simulink model "aIEEE13bus_with_solar_13bus_pl_1day"  (R2025a)
settings: Solver=ode4  StartTime=0.0  StopTime=168  FixedStep=5e-6  MaxStep=1e-4  RelTol=1e-4
InitFcn:
  | a=1; % Loading Factor
  | Ts=50e-6;
  | % phase to sequence conversion of RXB matrices
  | c=1*exp(sqrt(-1)*(120*pi/180));
  | T=[1 1 1;1 c*c c;1 c c*c];
  | Tinv=1/3*[1 1 1;1 c c*c;1 c*c c];
  | 
  | % Simulation data for the IEEE 13 Node Test Feeder model
  | mi2km = 1.60934;%  miles to km conversion
  | ft2km = 0.0003048; % feet to km conversion
  | ms2F = 1*1e-6/(2*pi*60);% microsiemens to Farads conversion
  | 
  | 
  | %% Configuration 601
  | % Series Resitance and Reactance - ohm/mile
  | R_601 = [0.3465 0.1560 0.1580;0.1560 0.3375 0.1535;0.1580 0.1535 0.3414];
  | X_601 = [1.1079 0.5017 0.4236;0.5017 1.0478 0.3849;0.4236 0.3849 1.0348];
  | % charging susceptance - microsiemens/mile
  | B_601 = [6.2998 -1.9958 -1.2595;-1.9958 5.9597 -0.7417;-1.2595 -0.7417 5.6386];
  | 
  | R_601 = R_601/mi2km;
  | Rseq=Tinv*R_601*T;
  | R1_601=Rseq(2,2);R0_601=Rseq(1,1);
  | 
  | L_601 = (X_601/(2*pi*60))/mi2km;
  | Lseq=Tinv*L_601*T;
  | L1_601=Lseq(2,2);L0_601=Lseq(1,1);
  | 
  | C_601 =(B_601*ms2F)/mi2km;
  | Cseq=Tinv*C_601*T;
  | C1_601=Cseq(2,2);C0_601=Cseq(1,1);
  | 
  | %% Configuration 602 - series reactance - ohm/mile
  | R_602 = [0.7526 0.1580 0.1560;0.1580 0.7475 0.1535;0.1560 0.1535 0.7436];
  | X_602 = [1.1814 0.4236 0.5017;0.4236 1.1983 0.3849;0.5017 0.3849 1.2112];
  | % charging susceptance - microsiemens/mile
  | B_602 = [5.6990 -1.0817 -1.6905;-1.0817 5.1795 -0.6588;-1.6905 -0.6588 5.4246];
  | 
  | R_602 = R_602/mi2km;
  | Rseq=Tinv*R_602*T;
  | R1_602=Rseq(2,2);R0_602=Rseq(1,1);
  | 
  | L_602 = (X_602/(2*pi*60))/mi2km;
  | Lseq=Tinv*L_602*T;
  | L1_602=Lseq(2,2);L0_602=Lseq(1,1);
  | 
  | C_602 =(B_602*ms2F)/mi2km;
  | Cseq=Tinv*C_602*T;
  | C1_602=Cseq(2,2);C0_602=Cseq(1,1);
  | %% Configuration 603 - series reactance - ohm/mile
  | R_603 = [0 0 0;0 1.3294 0.2066;0 0.2066 1.3238];
  | X_603 = [0 0 0;0 1.3471 0.4591;0 0.4591 1.3569];
  | % charging susceptance - microsiemens/mile
  | B_603 = [0 0 0;0 4.7097 -0.8999;0 -0.8999 4.6658];
  | 
  | % convert for SPS
  | R_603 = R_603/mi2km;
  | Rseq=Tinv*R_603*T;
  | R1_603=Rseq(2,2);R0_603=Rseq(1,1);
  | 
  | L_603 = (X_603/(2*pi*60))/mi2km;
  | Lseq=Tinv*L_603*T;
  | L1_603=Lseq(2,2);L0_603=Lseq(1,1);
  | 
  | C_603 =(B_603*ms2F)/mi2km;
  | Cseq=Tinv*C_603*T;
  | C1_603=Cseq(2,2);C0_603=Cseq(1,1);
  | %% Configuration 604 - series reactance - ohm/mile
  | R_604 = [1.3238 0 0.2066;0 0 0;0.2066 0 1.3294];
  | X_604 = [1.3569 0 0.4591;0 0 0;0.4591 0 1.3471];
  | % charging susceptance - microsiemens/mile
  | B_604 = [4.6658 0 -0.8999;0 0 0;-0.8999 0 4.7097];
  | R_604 = R_604/mi2km;
  | Rseq=Tinv*R_604*T;
  | R1_604=Rseq(2,2);R0_604=Rseq(1,1);
  | 
  | L_604 = (X_604/(2*pi*60))/mi2km;
  | Lseq=Tinv*L_604*T;
  | L1_604=Lseq(2,2);L0_604=Lseq(1,1);
  | 
  | C_604 =(B_604*ms2F)/mi2km;
  | Cseq=Tinv*C_604*T;
  | C1_604=Cseq(2,2);C0_604=Cseq(1,1);
  | %% Configuration 605 - series reactance - ohm/mile
  | R_605 = [0 0 0;0 0 0;0 0 1.3292];
  | X_605 = [0 0 0;0 0 0;0 0 1.3475];
  | % charging susceptance - microsiemens/mile
  | B_605 = [0 0 0;0 0 0;0 0 4.5193];
  | R_605 = R_605/mi2km;
  | Rseq=Tinv*R_605*T;
  | R1_605=Rseq(2,2);R0_605=Rseq(1,1);
  | 
  | L_605 = (X_605/(2*pi*60))/mi2km;
  | Lseq=Tinv*L_605*T;
  | L1_605=Lseq(2,2);L0_605=Lseq(1,1);
  | 
  | C_605 =(B_605*ms2F)/mi2km;
  | Cseq=Tinv*C_605*T;
  | C1_605=Cseq(2,2);C0_605=Cseq(1,1);
  | %% Configuration 606 - series reactance - ohm/mile
  | R_606 = [0.7982 0.3192 0.2849;0.3192 0.7891 0.3192;0.2849 0.3192 0.7982];
  | X_606 = [0.4463 0.0328 0.0143;0.0328 0.4041 0.0328;0.0143 0.0328 0.4463];
  | % charging susceptance - microsiemens/mile
  | B_606 = [96.8897 -1e-6 -1e-6;-1e-6 96.8897 -1e-6;-1e-6 -1e-6 96.8897];
  | R_606 = R_606/mi2km;
  | Rseq=Tinv*R_606*T;
  | R1_606=Rseq(2,2);R0_606=Rseq(1,1);
  | 
  | L_606 = (X_606/(2*pi*60))/mi2km;
  | Lseq=Tinv*L_606*T;
  | L1_606=Lseq(2,2);L0_606=Lseq(1,1);
  | 
  | C_606 =(B_606*ms2F)/mi2km;
  | Cseq=Tinv*C_606*T;
  | C1_606=Cseq(2,2);C0_606=Cseq(1,1);
  | %% Configuration 607 - series reactance - ohm/mile
  | R_607 = [1.3425 0 0;0 0 0;0 0 0];
  | X_607 = [0.5124 0 0;0 0 0;0 0 0];
  | % charging susceptance - microsiemens/mile
  | B_607 = [88.9912 0 0;0 0 0;0 0 0];
  | R_607 = R_607/mi2km;
  | Rseq=Tinv*R_607*T;
  | R1_607=Rseq(2,2);R0_607=Rseq(1,1);
  | 
  | L_607 = (X_607/(2*pi*60))/mi2km;
  | Lseq=Tinv*L_607*T;
  | L1_607=Lseq(2,2);L0_607=Lseq(1,1);
  | 
  | C_607 =(B_607*ms2F)/mi2km;
  | Cseq=Tinv*C_607*T;
  | C1_607=Cseq(2,2);C0_607=Cseq(1,1);
undefined symbols (not defined in the file or in its folder): D1, Delta, find_system, gcbh, sps_rtmsupport, Ts_Control, Ts_Power
libraries: spsSeriesRLCBranchLib x93, spsGroundLib x57, spsVoltageMeasurementLib x52, spsFourierLib x30, spsThreePhaseVIMeasurementLib x28, spsControlledCurrentSourceLib x25, spsVIMeasurementModel x21, slpidlib x16, spsabctodq0Lib x16, spsCurrentMeasurementLib x11, spsPower3phPhasorLib x11, spsThreePhaseSeriesRLCLoadLib x9
(part 1 of 9)
settings Model: ARTEMISmethode_block_infos=$$__separator__$$pi34variableloadwith3PV/ARTEMIS Guide$$__separator__$$  Creator=Arun  LastModifiedBy=Uttam Krishnan
settings SolverCC: ShapePreserveControl=EnableAll  AlgebraicLoopSolver=TrustRegion  SolverResetMethod=Robust
settings DataIOCC: ReturnWorkspaceOutputs=off
settings DebuggingCC: ArithmeticOperatorsInVariantConditions=warning
settings ModelReferenceCC: EnableRefExpFcnMdlSchedulingChecks=on
settings SFSimCC: SimUseLocalCustomCode=off  CustomCodeUndefinedFunction=UseInterfaceOnly
settings RTWCC: RTWUseLocalCustomCode=off  GPUComputeCapability=3.5
settings CodeAppCC: StateflowObjectComments=on
settings SimscapeCC: SimscapeNormalizeSystem=off

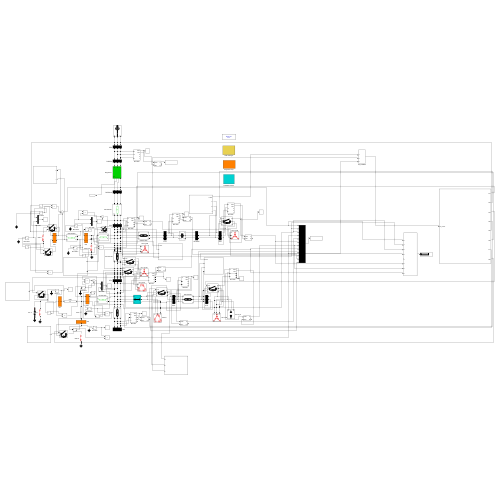
[thumbnail: Simulink's stored preview of the top-level diagram]
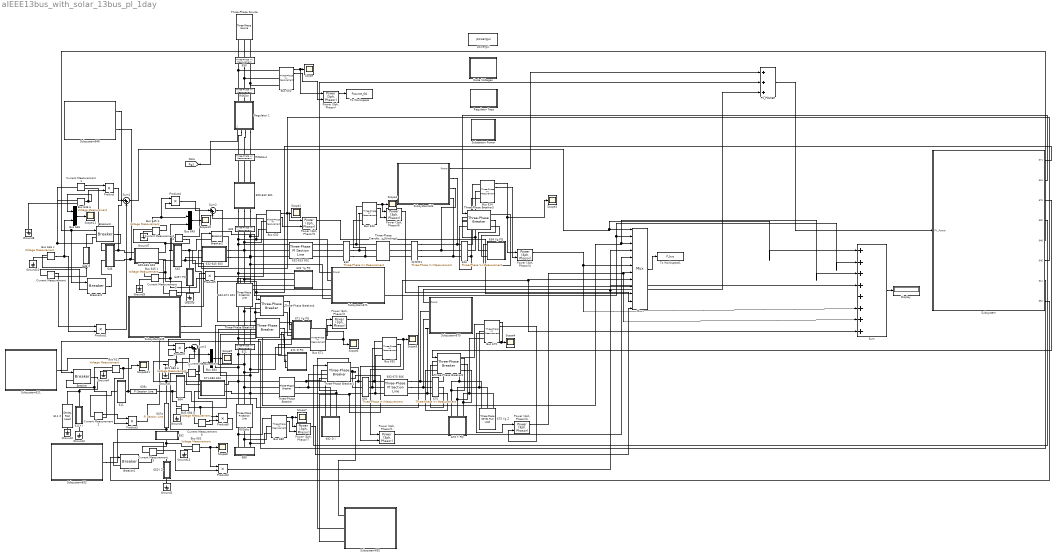
== system aIEEE13bus_with_solar_13bus_pl_1day ==
  601abc : spsThreePhasePISectionLineLib/Three-Phase PI Section Line  LConnTagsString=a|b|c  RConnTagsString=A|B|C  Length=1000*ft2km  Frequency=60  Resistances=[R1_601 R0_601]  Inductances=[L1_601 L0_601]  Capacitances=[C1_601 C0_601]
  605c : spsPiSectionLineLib/Pi Section Line  LConnTagsString=__new0  RConnTagsString=__new0  Phases=1  PiSections=1  Length=300*ft2km  Frequency=60  Resistance=R1_605  Inductance=L1_605  Capacitance=C1_605  SpecifyConductance=off  Conductance=0  Measurements=None  Measurements2=None
  607a : spsPiSectionLineLib/Pi Section Line  LConnTagsString=__new0  RConnTagsString=__new0  Phases=1  PiSections=1  Length=800*ft2km  Frequency=60  Resistance=R1_607  Inductance=L1_607  Capacitance=C1_607  SpecifyConductance=off  Conductance=0  Measurements=None  Measurements2=None
  611 : Subsystem
  611 Z : spsSeriesRLCLoadLib/Series RLC Load  LConnTagsString=a  RConnTagsString=__new0  NominalVoltage=2401.78  NominalFrequency=60  ActivePower=0  InductivePower=0  CapacitivePower=100e3*a  Setx0=off  InitialVoltage=0  SetiL0=off  InitialCurrent=0  Measurements=None  LoadType=constant Z
  611Y I : Subsystem  mask(Single Phase ZIP Load){Vnom=1*2401.78, fnom=60, Pnom=170e3*a, Qnom=80e3*a, LoadType=constant I, Vlim=0.7}
      mask prompts: Vnom "Nominal Voltage Vn (Vrms)"; fnom "Nominal Frequency fn (Hz)"; Pnom "Nominal Active power (W)"; Qnom "Nominal Reactive power (VAR)"; LoadType "Load Type"; Vlim "Minimum voltage (pu)"
      mask help:
      | Notes:
      | Single Phase ZIP load model which gets converted to constant Z type if the voltage becomes lower than the "Minimum voltage".
      mask TypeOptions LoadType: Constant Z | constant I | constant P
      mask DialogControl ParameterTabVar0 Prompt: Parameters
      mask DialogControl ParameterTabVar1 Prompt: Type
      mask Display:
      | color('red');
      | A=[-210,-180,-170,-160,-147,-140,-130,-120,-110,-80,-50,-49,-45,-39,-33,-26,-21,-18,-17,-19,-22,-22,-26,-27,-25,-22,-16,-9,-3,2,6,6,4,1,1,-3,-4,-2,2,7,14,20,26,29,30,28,24,24,21,20,21,25,31,37,44,49,50,50,80];
      | B=[-41.5,-41.5,-63,-20,-63,-20,-63,-20,-41.5,-41.5,-41.5,-34,-26,-21,-20,-22,-28,-37,-47,-57,-63,-63,-54,-44,-34,-26,-21,-20,-22,-28,-37,-47,-57,-63,-63,-54,-44,-34,-26,-21,-20,-22,-28,-37,-47,-57,-63,-63,-54,-44,-34,-26,-21,-20,-22,-28,-37,-41.50,-41.5];
      | plot(A,B);
      | color('black');
      | port_label('LConn', 1, '+')
  632 : spsThreePhaseVIMeasurementLib/Three-Phase V-I Measurement  VoltageMeasurement=phase-to-ground  SetLabelV=on  LabelV=V632  Vpu=off  VpuLL=off  CurrentMeasurement=yes  SetLabelI=on  LabelI=I632  Ipu=off  Pbase=100e6  Vbase=24900  OutputType=Complex  PhasorSimulation=off  PSBequivalent=0
  632 Yg PQ : Subsystem  mask(Three Phase Star ZIP Load (Phasor)){Vnom=4160, fnom=60, Pnom=[17 66  117]*1e3/4*a, Qnom=[10 38  68]*1e3/4*a, LoadType=Constant P, Vlim=0.7}
      mask prompts: Vnom "Nominal Ph-Ph voltage (Vrms)"; fnom "Nominal Frequency fn (Hz)"; Pnom "Nominal Per Phase Active Power [Pa Pb Pc] (W)"; Qnom "Nominal Per Phase Reactive Power [Qa Qb Qc] (VAR)"; LoadType "Load Type"; Vlim "Minimum voltage (pu)"
      mask help:
      | Notes:
      | Three Phase Star Connected ZIP load model which gets converted to constant Z type if the voltage becomes lower than the "Minimum voltage".
      mask TypeOptions LoadType: Constant Z | Constant I | Constant P
      mask DialogControl ParameterTabVar0 Prompt: Parameters
      mask DialogControl ParameterTabVar01 Prompt: Type
      mask Display:
      | color('red');
      | %load figure 0deg
      | A=[-210,-180,-170,-160,-147,-140,-130,-120,-110,-80,-50,-49,-45,-39,-33,-26,-21,-18,-17,-19,-22,-22,-26,-27,-25,-22,-16,-9,-3,2,6,6,4,1,1,-3,-4,-2,2,7,14,20,26,29,30,28,24,24,21,20,21,25,31,37,44,49,50,50,80];
      | B=[-41.5,-41.5,-63,-20,-63,-20,-63,-20,-41.5,-41.5,-41.5,-34,-26,-21,-20,-22,-28,-37,-47,-57,-63,-63,-54,-44,-34,-26,-21,-20,-22,-28,-37,-47,-57,-63,-63,-54,-44,-34,-26,-21,-20,-22,-28,-37,-47,-57,-63,-63,-54,-44,-34,-26,-21,-20,-22,-28,-37,-41.50,-41.5];
      | % plot(A,B);
      | 
      | %load figure 0deg inverted
      | A1=[-80,-50,-49,-45,-39,-33,-26,-21,-18,-17,-19,-22,-22,-26,-27,-25,-22,-16,-9,-3,2,6,6,4,1,1,-3,-4,-2,2,7,14,20,26,29,30,28,24,24,21,20,21,25,31,37,44,49,50,50,80,110,120,130,143,150,160,170,180,210];
      | B1=[-41.5,-41.5,-34,-26,-21,-20,-22,-28,-37,-47,-57,-63,-63,-54,-44,-34,-26,-21,-20,-22,-28,-37,-47,-57,-63,-63,-54,-44,-34,-26,-21,-20,-22,-28,-37,-47,-57,-63,-63,-54,-44,-34,-26,-21,-20,-22,-28,-37,-41.5,-41.5,-41.5,-63,-20,-63,-20,-63,-20,-41.5,-41.5];
      | 
      | 
      | %load figure 90deg
      | C=[-41.5,-41.5,-20,-63,-20,-63,-20,-63,-41.5,-41.5,-41.5,-37,-28,-22,-20,-21,-26,-34,-44,-54,-63,-63,-57,-47,-37,-28,-22,-20,-21,-26,-34,-44,-54,-63,-63,-57,-47,-37,-28,-22,-20,-21,-26,-34,-44,-54,-63,-63,-57,-47,-37,-28,-22,-20,-21,-26,-34,-41.5,-41.5];
      | D=[190,160,150,140,130,123,110,100,90,80,50,50,49,44,37,31,25,21,20,21,24,24,28,30,29,26,20,14,7,2,-2,-4,-3,1,1,4,6,6,2,-3,-9,-16,-22,-25,-27,-26,-22,-22,-19,-17,-18,-21,-26,-33,-39,-45,-49,-50,-70];
      | plot(C,D);
      | 
      | 
      | %load figure -120deg
      | c=1*exp(sqrt(-1)*(-60*pi/180));
      | l=A1+j*B1;
      | m=l*c;
      | E=real(m);F=imag(m);
      | E=E+34.4400;F=F-118.53;
      | plot(E,F);
      | 
      | %load figure +120deg
      | c=1*exp(sqrt(-1)*(60*pi/180));
      | l=A+j*B;
      | m=l*c;
      | G=real(m);
      | H=imag(m);
      | G=G-117.44;H=H-118.5300;
      | plot(G,H);
      | 
      | color('black');
      | port_label('LConn', 1, 'A')
      | port_label('LConn', 2, 'B')
      | port_label('LConn', 3, 'C')
  632-633 602 : spsThreePhasePISectionLineLib/Three-Phase PI Section Line  LConnTagsString=a|b|c  RConnTagsString=A|B|C  Length=500*ft2km  Frequency=60  Resistances=[R1_602 R0_602]  Inductances=[L1_602 L0_602]  Capacitances=[C1_602 C0_602]
  632-645 603 : Subsystem  mask(Two-Phase PI Section Block){Rl=R_603, Ll=L_603, Cl=C_603, L=500*ft2km}
      mask prompts: Rl "Resistance per unit Length(Ohm/Km)[3x3 matrix]"; Ll "Inductance per unit Length(H/Km)[3x3 matrix]"; Cl "Capacitance per unit Length(F/Km)[3x3 matrix"; L "Length (Km)"
      mask help: This block models a two-phase transmission line with a single PI section.
      mask init:
      | W = sign(sum(abs(Rl)));
      | s = find(W==1);%Identify non zero rows and columns
      | 
      | Rt =Rl(s,s);
      | Rl= Rt;
      | Lt =Ll(s,s);
      | Ll= Lt;
      | Ct =Cl(s,s);
      | Cl= Ct;
      mask Display:
      | color('green')
      | plot(0,0,100,100,[20,20,80,80,90,80,80,20,20,10],[50,40,40,50,50,50,61,61,50,50],[56,39],[55,55],[44,44],[44,55],[53,50,50],[44,48,55])
      | color('black')
      | port_label('RConn', 1, 'b')
      | port_label('RConn', 2, 'c')
      | port_label('LConn', 1, 'B')
      | port_label('LConn', 2, 'C')
  632-671 601 : spsThreePhasePISectionLineLib/Three-Phase PI Section Line  LConnTagsString=a|b|c  RConnTagsString=A|B|C  Length=2000*ft2km  Frequency=60  Resistances=[R1_601 R0_601]  Inductances=[L1_601 L0_601]  Capacitances=[C1_601 C0_601]
  633 : spsThreePhaseVIMeasurementLib/Three-Phase V-I Measurement  VoltageMeasurement=phase-to-ground  SetLabelV=on  LabelV=V633  Vpu=off  VpuLL=off  CurrentMeasurement=no  SetLabelI=on  LabelI=I634  Ipu=off  Pbase=100e6  Vbase=24900  OutputType=Complex  PhasorSimulation=off  PSBequivalent=0
  634 : spsThreePhaseVIMeasurementLib/Three-Phase V-I Measurement  VoltageMeasurement=phase-to-ground  SetLabelV=on  LabelV=V634  Vpu=off  VpuLL=off  CurrentMeasurement=yes  SetLabelI=on  LabelI=I634  Ipu=off  Pbase=100e6  Vbase=24900  OutputType=Complex  PhasorSimulation=off  PSBequivalent=0
  634 Yg PQ : Subsystem  mask(Three Phase Star ZIP Load (Phasor)){Vnom=480, fnom=60, Pnom=[160 120 120]*1e3*a, Qnom=[110 90 90]*1e3*a, LoadType=Constant P, Vlim=0.7}
      mask prompts: Vnom "Nominal Ph-Ph voltage (Vrms)"; fnom "Nominal Frequency fn (Hz)"; Pnom "Nominal Per Phase Active Power [Pa Pb Pc] (W)"; Qnom "Nominal Per Phase Reactive Power [Qa Qb Qc] (VAR)"; LoadType "Load Type"; Vlim "Minimum voltage (pu)"
      mask help:
      | Notes:
      | Three Phase Star Connected ZIP load model which gets converted to constant Z type if the voltage becomes lower than the "Minimum voltage".
      mask TypeOptions LoadType: Constant Z | Constant I | Constant P
      mask DialogControl ParameterTabVar0 Prompt: Parameters
      mask DialogControl ParameterTabVar01 Prompt: Type
      mask Display:
      | color('red');
      | %load figure 0deg
      | A=[-210,-180,-170,-160,-147,-140,-130,-120,-110,-80,-50,-49,-45,-39,-33,-26,-21,-18,-17,-19,-22,-22,-26,-27,-25,-22,-16,-9,-3,2,6,6,4,1,1,-3,-4,-2,2,7,14,20,26,29,30,28,24,24,21,20,21,25,31,37,44,49,50,50,80];
      | B=[-41.5,-41.5,-63,-20,-63,-20,-63,-20,-41.5,-41.5,-41.5,-34,-26,-21,-20,-22,-28,-37,-47,-57,-63,-63,-54,-44,-34,-26,-21,-20,-22,-28,-37,-47,-57,-63,-63,-54,-44,-34,-26,-21,-20,-22,-28,-37,-47,-57,-63,-63,-54,-44,-34,-26,-21,-20,-22,-28,-37,-41.50,-41.5];
      | % plot(A,B);
      | 
      | %load figure 0deg inverted
      | A1=[-80,-50,-49,-45,-39,-33,-26,-21,-18,-17,-19,-22,-22,-26,-27,-25,-22,-16,-9,-3,2,6,6,4,1,1,-3,-4,-2,2,7,14,20,26,29,30,28,24,24,21,20,21,25,31,37,44,49,50,50,80,110,120,130,143,150,160,170,180,210];
      | B1=[-41.5,-41.5,-34,-26,-21,-20,-22,-28,-37,-47,-57,-63,-63,-54,-44,-34,-26,-21,-20,-22,-28,-37,-47,-57,-63,-63,-54,-44,-34,-26,-21,-20,-22,-28,-37,-47,-57,-63,-63,-54,-44,-34,-26,-21,-20,-22,-28,-37,-41.5,-41.5,-41.5,-63,-20,-63,-20,-63,-20,-41.5,-41.5];
      | 
      | 
      | %load figure 90deg
      | C=[-41.5,-41.5,-20,-63,-20,-63,-20,-63,-41.5,-41.5,-41.5,-37,-28,-22,-20,-21,-26,-34,-44,-54,-63,-63,-57,-47,-37,-28,-22,-20,-21,-26,-34,-44,-54,-63,-63,-57,-47,-37,-28,-22,-20,-21,-26,-34,-44,-54,-63,-63,-57,-47,-37,-28,-22,-20,-21,-26,-34,-41.5,-41.5];
      | D=[190,160,150,140,130,123,110,100,90,80,50,50,49,44,37,31,25,21,20,21,24,24,28,30,29,26,20,14,7,2,-2,-4,-3,1,1,4,6,6,2,-3,-9,-16,-22,-25,-27,-26,-22,-22,-19,-17,-18,-21,-26,-33,-39,-45,-49,-50,-70];
      | plot(C,D);
      | 
      | 
      | %load figure -120deg
      | c=1*exp(sqrt(-1)*(-60*pi/180));
      | l=A1+j*B1;
      | m=l*c;
      | E=real(m);F=imag(m);
      | E=E+34.4400;F=F-118.53;
      | plot(E,F);
      | 
      | %load figure +120deg
      | c=1*exp(sqrt(-1)*(60*pi/180));
      | l=A+j*B;
      | m=l*c;
      | G=real(m);
      | H=imag(m);
      | G=G-117.44;H=H-118.5300;
      | plot(G,H);
      | 
      | color('black');
      | port_label('LConn', 1, 'A')
      | port_label('LConn', 2, 'B')
      | port_label('LConn', 3, 'C')
  645 : Subsystem
  645-646 603 : Subsystem  mask(Two-Phase PI Section Block){Rl=R_603, Ll=L_603, Cl=C_603, L=300*ft2km}
      mask prompts: Rl "Resistance per unit Length(Ohm/Km)[3x3 matrix]"; Ll "Inductance per unit Length(H/Km)[3x3 matrix]"; Cl "Capacitance per unit Length(F/Km)[3x3 matrix"; L "Length (Km)"
      mask help: This block models a two-phase transmission line with a single PI section.
      mask init:
      | W = sign(sum(abs(Rl)));
      | s = find(W==1);%Identify non zero rows and columns
      | 
      | Rt =Rl(s,s);
      | Rl= Rt;
      | Lt =Ll(s,s);
      | Ll= Lt;
      | Ct =Cl(s,s);
      | Cl= Ct;
      mask Display:
      | color('green')
      | plot(0,0,100,100,[20,20,80,80,90,80,80,20,20,10],[50,40,40,50,50,50,61,61,50,50],[56,39],[55,55],[44,44],[44,55],[53,50,50],[44,48,55])
      | color('black')
      | port_label('RConn', 1, 'b')
      | port_label('RConn', 2, 'c')
      | port_label('LConn', 1, 'B')
      | port_label('LConn', 2, 'C')
  645Y PQ : Subsystem  mask(Single Phase ZIP Load){Vnom=1*2401.78, fnom=60, Pnom=170e3*a, Qnom=125e3*a, LoadType=constant P, Vlim=0.7}
      mask prompts: Vnom "Nominal Voltage Vn (Vrms)"; fnom "Nominal Frequency fn (Hz)"; Pnom "Nominal Active power (W)"; Qnom "Nominal Reactive power (VAR)"; LoadType "Load Type"; Vlim "Minimum voltage (pu)"
      mask help:
      | Notes:
      | Single Phase ZIP load model which gets converted to constant Z type if the voltage becomes lower than the "Minimum voltage".
      mask TypeOptions LoadType: Constant Z | constant I | constant P
      mask DialogControl ParameterTabVar0 Prompt: Parameters
      mask DialogControl ParameterTabVar1 Prompt: Type
      mask Display:
      | color('red');
      | A=[-210,-180,-170,-160,-147,-140,-130,-120,-110,-80,-50,-49,-45,-39,-33,-26,-21,-18,-17,-19,-22,-22,-26,-27,-25,-22,-16,-9,-3,2,6,6,4,1,1,-3,-4,-2,2,7,14,20,26,29,30,28,24,24,21,20,21,25,31,37,44,49,50,50,80];
      | B=[-41.5,-41.5,-63,-20,-63,-20,-63,-20,-41.5,-41.5,-41.5,-34,-26,-21,-20,-22,-28,-37,-47,-57,-63,-63,-54,-44,-34,-26,-21,-20,-22,-28,-37,-47,-57,-63,-63,-54,-44,-34,-26,-21,-20,-22,-28,-37,-47,-57,-63,-63,-54,-44,-34,-26,-21,-20,-22,-28,-37,-41.50,-41.5];
      | plot(A,B);
      | color('black');
      | port_label('LConn', 1, '+')
  646 : Subsystem
  646 Z : Subsystem  mask(Single Phase ZIP Load){Vnom=4160, fnom=60, Pnom=230e3*a, Qnom=132e3*a, LoadType=Constant Z, Vlim=0.7}
      mask prompts: Vnom "Nominal Voltage Vn (Vrms)"; fnom "Nominal Frequency fn (Hz)"; Pnom "Nominal Active power (W)"; Qnom "Nominal Reactive power (VAR)"; LoadType "Load Type"; Vlim "Minimum voltage (pu)"
      mask help:
      | Notes:
      | Single Phase ZIP load model which gets converted to constant Z type if the voltage becomes lower than the "Minimum voltage".
      mask TypeOptions LoadType: Constant Z | constant I | constant P
      mask DialogControl ParameterTabVar0 Prompt: Parameters
      mask DialogControl ParameterTabVar1 Prompt: Type
      mask Display:
      | color('red');
      | A=[-210,-180,-170,-160,-147,-140,-130,-120,-110,-80,-50,-49,-45,-39,-33,-26,-21,-18,-17,-19,-22,-22,-26,-27,-25,-22,-16,-9,-3,2,6,6,4,1,1,-3,-4,-2,2,7,14,20,26,29,30,28,24,24,21,20,21,25,31,37,44,49,50,50,80];
      | B=[-41.5,-41.5,-63,-20,-63,-20,-63,-20,-41.5,-41.5,-41.5,-34,-26,-21,-20,-22,-28,-37,-47,-57,-63,-63,-54,-44,-34,-26,-21,-20,-22,-28,-37,-47,-57,-63,-63,-54,-44,-34,-26,-21,-20,-22,-28,-37,-47,-57,-63,-63,-54,-44,-34,-26,-21,-20,-22,-28,-37,-41.50,-41.5];
      | plot(A,B);
      | color('black');
      | port_label('LConn', 1, '+')
  650 : spsThreePhaseVIMeasurementLib/Three-Phase V-I Measurement  VoltageMeasurement=phase-to-ground  SetLabelV=on  LabelV=V650  Vpu=off  VpuLL=off  CurrentMeasurement=yes  SetLabelI=on  LabelI=I650  Ipu=off  Pbase=100e6  Vbase=24900  OutputType=Complex  PhasorSimulation=off  PSBequivalent=0
  650-632 601 : Subsystem  mask(Three-Phase PI Section Block){Rl=R_601, Ll=L_601, Cl=C_601, L=2000*ft2km}
      mask prompts: Rl "Resistance per unit Length(Ohm/Km)[3x3 matrix]"; Ll "Inductance per unit Length(H/Km)[3x3 matrix]"; Cl "Capacitance per unit Length(F/Km)[3x3 matrix]"; L "Length (Km)"
      mask help: This block models a three-phase transmission line with a single PI section.
      mask Display:
      | color('green')
      | plot(0,0,100,100,[20,20,80,80,90,80,80,20,20,10],[50,40,40,50,50,50,61,61,50,50],[56,39],[55,55],[44,44],[44,55],[53,50,50],[44,48,55])
      | color('black')
      | port_label('RConn', 1, 'a')
      | port_label('RConn', 2, 'b')
      | port_label('RConn', 3, 'c')
      | port_label('LConn', 1, 'A')
      | port_label('LConn', 2, 'B')
      | port_label('LConn', 3, 'C')
  652 : Subsystem
  652Y Z : Subsystem  mask(Single Phase ZIP Load){Vnom=1.0*2401.78, fnom=60, Pnom=128e3*a, Qnom=86e3*a, LoadType=Constant Z, Vlim=0.7}
      mask prompts: Vnom "Nominal Voltage Vn (Vrms)"; fnom "Nominal Frequency fn (Hz)"; Pnom "Nominal Active power (W)"; Qnom "Nominal Reactive power (VAR)"; LoadType "Load Type"; Vlim "Minimum voltage (pu)"
      mask help:
      | Notes:
      | Single Phase ZIP load model which gets converted to constant Z type if the voltage becomes lower than the "Minimum voltage".
      mask TypeOptions LoadType: Constant Z | constant I | constant P
      mask DialogControl ParameterTabVar0 Prompt: Parameters
      mask DialogControl ParameterTabVar1 Prompt: Type
      mask Display:
      | color('red');
      | A=[-210,-180,-170,-160,-147,-140,-130,-120,-110,-80,-50,-49,-45,-39,-33,-26,-21,-18,-17,-19,-22,-22,-26,-27,-25,-22,-16,-9,-3,2,6,6,4,1,1,-3,-4,-2,2,7,14,20,26,29,30,28,24,24,21,20,21,25,31,37,44,49,50,50,80];
      | B=[-41.5,-41.5,-63,-20,-63,-20,-63,-20,-41.5,-41.5,-41.5,-34,-26,-21,-20,-22,-28,-37,-47,-57,-63,-63,-54,-44,-34,-26,-21,-20,-22,-28,-37,-47,-57,-63,-63,-54,-44,-34,-26,-21,-20,-22,-28,-37,-47,-57,-63,-63,-54,-44,-34,-26,-21,-20,-22,-28,-37,-41.50,-41.5];
      | plot(A,B);
      | color('black');
      | port_label('LConn', 1, '+')
  671 : spsThreePhaseVIMeasurementLib/Three-Phase V-I Measurement  VoltageMeasurement=phase-to-ground  SetLabelV=on  LabelV=V671  Vpu=off  VpuLL=off  CurrentMeasurement=no  SetLabelI=on  LabelI=I634  Ipu=off  Pbase=100e6  Vbase=24900  OutputType=Complex  PhasorSimulation=off  PSBequivalent=0
  671 D PQ : Subsystem  mask(Three Phase Delta ZIP Load (Phasor)){Vnom=4160, fnom=60, Pnom=[385 385 385 ]*1e3*a, Qnom=[220 220 220]*1e3*a, LoadType=Constant P, Vlim=0.7}
      mask prompts: Vnom "Nominal Ph-Ph Voltage (Vrms)"; fnom "Nominal Frequency fn (Hz)"; Pnom "Nominal Per Phase Active Power [Pab Pbc Pca] (W)"; Qnom "Nominal Per Phase Reactive Power [Qab Qbc Qca] (VAR)"; LoadType "Load Type"; Vlim "Minimum Voltage (pu)"
      mask help:
      | Notes:
      | Three Phase Delta Connected ZIP load model which gets converted to constant Z type if the voltage becomes lower than the "Minimum voltage".
      mask TypeOptions LoadType: Constant Z | Constant I | Constant P
      mask DialogControl ParameterTabVar0 Prompt: Parameters
      mask DialogControl ParameterTabVar01 Prompt: Type
      mask Display:
      | color('red');
      | %load figure 0deg
      | A=[-210,-180,-170,-160,-147,-140,-130,-120,-110,-80,-50,-49,-45,-39,-33,-26,-21,-18,-17,-19,-22,-22,-26,-27,-25,-22,-16,-9,-3,2,6,6,4,1,1,-3,-4,-2,2,7,14,20,26,29,30,28,24,24,21,20,21,25,31,37,44,49,50,50,80];
      | B=[-41.5,-41.5,-63,-20,-63,-20,-63,-20,-41.5,-41.5,-41.5,-34,-26,-21,-20,-22,-28,-37,-47,-57,-63,-63,-54,-44,-34,-26,-21,-20,-22,-28,-37,-47,-57,-63,-63,-54,-44,-34,-26,-21,-20,-22,-28,-37,-47,-57,-63,-63,-54,-44,-34,-26,-21,-20,-22,-28,-37,-41.50,-41.5];
      | plot(A,B);
      | 
      | %load figure 0deg inverted
      | A1=[-80,-50,-49,-45,-39,-33,-26,-21,-18,-17,-19,-22,-22,-26,-27,-25,-22,-16,-9,-3,2,6,6,4,1,1,-3,-4,-2,2,7,14,20,26,29,30,28,24,24,21,20,21,25,31,37,44,49,50,50,80,110,120,130,143,150,160,170,180,210];
      | B1=[-41.5,-41.5,-34,-26,-21,-20,-22,-28,-37,-47,-57,-63,-63,-54,-44,-34,-26,-21,-20,-22,-28,-37,-47,-57,-63,-63,-54,-44,-34,-26,-21,-20,-22,-28,-37,-47,-57,-63,-63,-54,-44,-34,-26,-21,-20,-22,-28,-37,-41.5,-41.5,-41.5,-63,-20,-63,-20,-63,-20,-41.5,-41.5];
      | 
      | 
      | %load figure -120deg
      | c=1*exp(sqrt(-1)*(-60*pi/180));
      | l=A1+j*B1;
      | m=l*c;
      | E=real(m);F=imag(m);
      | E=E+10.94;F=F+161.1;
      | plot(E,F);
      | 
      | %load figure +120deg
      | c=1*exp(sqrt(-1)*(60*pi/180));
      | l=A1+j*B1;
      | m=l*c;
      | G=real(m);
      | H=imag(m);
      | G=G-205.94;H=H+48.53;
      | plot(G,H);
      | 
      | color('black');
      | port_label('LConn', 1, 'A')
      | port_label('LConn', 2, 'B')
      | port_label('LConn', 3, 'C')
  671 Yg PQ : Subsystem  mask(Three Phase Star ZIP Load (Phasor)){Vnom=4160, fnom=60, Pnom=3*[17 66  117]*1e3/4*a, Qnom=3*[10 38  68]*1e3/4*a, LoadType=Constant P, Vlim=0.7}
      mask prompts: Vnom "Nominal Ph-Ph voltage (Vrms)"; fnom "Nominal Frequency fn (Hz)"; Pnom "Nominal Per Phase Active Power [Pa Pb Pc] (W)"; Qnom "Nominal Per Phase Reactive Power [Qa Qb Qc] (VAR)"; LoadType "Load Type"; Vlim "Minimum voltage (pu)"
      mask help:
      | Notes:
      | Three Phase Star Connected ZIP load model which gets converted to constant Z type if the voltage becomes lower than the "Minimum voltage".
      mask TypeOptions LoadType: Constant Z | Constant I | Constant P
      mask DialogControl ParameterTabVar0 Prompt: Parameters
      mask DialogControl ParameterTabVar01 Prompt: Type
      mask Display:
      | color('red');
      | %load figure 0deg
      | A=[-210,-180,-170,-160,-147,-140,-130,-120,-110,-80,-50,-49,-45,-39,-33,-26,-21,-18,-17,-19,-22,-22,-26,-27,-25,-22,-16,-9,-3,2,6,6,4,1,1,-3,-4,-2,2,7,14,20,26,29,30,28,24,24,21,20,21,25,31,37,44,49,50,50,80];
      | B=[-41.5,-41.5,-63,-20,-63,-20,-63,-20,-41.5,-41.5,-41.5,-34,-26,-21,-20,-22,-28,-37,-47,-57,-63,-63,-54,-44,-34,-26,-21,-20,-22,-28,-37,-47,-57,-63,-63,-54,-44,-34,-26,-21,-20,-22,-28,-37,-47,-57,-63,-63,-54,-44,-34,-26,-21,-20,-22,-28,-37,-41.50,-41.5];
      | % plot(A,B);
      | 
      | %load figure 0deg inverted
      | A1=[-80,-50,-49,-45,-39,-33,-26,-21,-18,-17,-19,-22,-22,-26,-27,-25,-22,-16,-9,-3,2,6,6,4,1,1,-3,-4,-2,2,7,14,20,26,29,30,28,24,24,21,20,21,25,31,37,44,49,50,50,80,110,120,130,143,150,160,170,180,210];
      | B1=[-41.5,-41.5,-34,-26,-21,-20,-22,-28,-37,-47,-57,-63,-63,-54,-44,-34,-26,-21,-20,-22,-28,-37,-47,-57,-63,-63,-54,-44,-34,-26,-21,-20,-22,-28,-37,-47,-57,-63,-63,-54,-44,-34,-26,-21,-20,-22,-28,-37,-41.5,-41.5,-41.5,-63,-20,-63,-20,-63,-20,-41.5,-41.5];
      | 
      | 
      | %load figure 90deg
      | C=[-41.5,-41.5,-20,-63,-20,-63,-20,-63,-41.5,-41.5,-41.5,-37,-28,-22,-20,-21,-26,-34,-44,-54,-63,-63,-57,-47,-37,-28,-22,-20,-21,-26,-34,-44,-54,-63,-63,-57,-47,-37,-28,-22,-20,-21,-26,-34,-44,-54,-63,-63,-57,-47,-37,-28,-22,-20,-21,-26,-34,-41.5,-41.5];
      | D=[190,160,150,140,130,123,110,100,90,80,50,50,49,44,37,31,25,21,20,21,24,24,28,30,29,26,20,14,7,2,-2,-4,-3,1,1,4,6,6,2,-3,-9,-16,-22,-25,-27,-26,-22,-22,-19,-17,-18,-21,-26,-33,-39,-45,-49,-50,-70];
      | plot(C,D);
      | 
      | 
      | %load figure -120deg
      | c=1*exp(sqrt(-1)*(-60*pi/180));
      | l=A1+j*B1;
      | m=l*c;
      | E=real(m);F=imag(m);
      | E=E+34.4400;F=F-118.53;
      | plot(E,F);
      | 
      | %load figure +120deg
      | c=1*exp(sqrt(-1)*(60*pi/180));
      | l=A+j*B;
      | m=l*c;
      | G=real(m);
      | H=imag(m);
      | G=G-117.44;H=H-118.5300;
      | plot(G,H);
      | 
      | color('black');
      | port_label('LConn', 1, 'A')
      | port_label('LConn', 2, 'B')
      | port_label('LConn', 3, 'C')
  671-684 604 : Subsystem  mask(Two-Phase PI Section Block){Rl=R_604, Ll=L_604, Cl=C_604, L=300*ft2km}
      mask prompts: Rl "Resistance per unit Length(Ohm/Km)[3x3 matrix]"; Ll "Inductance per unit Length(H/Km)[3x3 matrix]"; Cl "Capacitance per unit Length(F/Km)[3x3 matrix"; L "Length (Km)"
      mask help: This block models a two-phase transmission line with a single PI section.
      mask init:
      | W = sign(sum(abs(Rl)));
      | s = find(W==1);%Identify non zero rows and columns
      | 
      | Rt =Rl(s,s);
      | Rl= Rt;
      | Lt =Ll(s,s);
      | Ll= Lt;
      | Ct =Cl(s,s);
      | Cl= Ct;
      mask Display:
      | color('green')
      | plot(0,0,100,100,[20,20,80,80,90,80,80,20,20,10],[50,40,40,50,50,50,61,61,50,50],[56,39],[55,55],[44,44],[44,55],[53,50,50],[44,48,55])
      | color('black')
      | port_label('RConn', 1, 'a')
      | port_label('RConn', 2, 'c')
      | port_label('LConn', 1, 'A')
      | port_label('LConn', 2, 'C')
  675 : spsThreePhaseVIMeasurementLib/Three-Phase V-I Measurement  VoltageMeasurement=phase-to-ground  SetLabelV=on  LabelV=V675  Vpu=off  VpuLL=off  CurrentMeasurement=no  SetLabelI=on  LabelI=I634  Ipu=off  Pbase=100e6  Vbase=24900  OutputType=Complex  PhasorSimulation=off  PSBequivalent=0
  675 Y PQ : Subsystem  mask(Three Phase Star ZIP Load (Phasor)){Vnom=4160, fnom=60, Pnom=[485  68  290]*1e3*a, Qnom=[190  60  212]*1e3*a, LoadType=Constant P, Vlim=0.7}
      mask prompts: Vnom "Nominal Ph-Ph voltage (Vrms)"; fnom "Nominal Frequency fn (Hz)"; Pnom "Nominal Per Phase Active Power [Pa Pb Pc] (W)"; Qnom "Nominal Per Phase Reactive Power [Qa Qb Qc] (VAR)"; LoadType "Load Type"; Vlim "Minimum voltage (pu)"
      mask help:
      | Notes:
      | Three Phase Star Connected ZIP load model which gets converted to constant Z type if the voltage becomes lower than the "Minimum voltage".
      mask TypeOptions LoadType: Constant Z | Constant I | Constant P
      mask DialogControl ParameterTabVar0 Prompt: Parameters
      mask DialogControl ParameterTabVar01 Prompt: Type
      mask Display:
      | color('red');
      | %load figure 0deg
      | A=[-210,-180,-170,-160,-147,-140,-130,-120,-110,-80,-50,-49,-45,-39,-33,-26,-21,-18,-17,-19,-22,-22,-26,-27,-25,-22,-16,-9,-3,2,6,6,4,1,1,-3,-4,-2,2,7,14,20,26,29,30,28,24,24,21,20,21,25,31,37,44,49,50,50,80];
      | B=[-41.5,-41.5,-63,-20,-63,-20,-63,-20,-41.5,-41.5,-41.5,-34,-26,-21,-20,-22,-28,-37,-47,-57,-63,-63,-54,-44,-34,-26,-21,-20,-22,-28,-37,-47,-57,-63,-63,-54,-44,-34,-26,-21,-20,-22,-28,-37,-47,-57,-63,-63,-54,-44,-34,-26,-21,-20,-22,-28,-37,-41.50,-41.5];
      | % plot(A,B);
      | 
      | %load figure 0deg inverted
      | A1=[-80,-50,-49,-45,-39,-33,-26,-21,-18,-17,-19,-22,-22,-26,-27,-25,-22,-16,-9,-3,2,6,6,4,1,1,-3,-4,-2,2,7,14,20,26,29,30,28,24,24,21,20,21,25,31,37,44,49,50,50,80,110,120,130,143,150,160,170,180,210];
      | B1=[-41.5,-41.5,-34,-26,-21,-20,-22,-28,-37,-47,-57,-63,-63,-54,-44,-34,-26,-21,-20,-22,-28,-37,-47,-57,-63,-63,-54,-44,-34,-26,-21,-20,-22,-28,-37,-47,-57,-63,-63,-54,-44,-34,-26,-21,-20,-22,-28,-37,-41.5,-41.5,-41.5,-63,-20,-63,-20,-63,-20,-41.5,-41.5];
      | 
      | 
      | %load figure 90deg
      | C=[-41.5,-41.5,-20,-63,-20,-63,-20,-63,-41.5,-41.5,-41.5,-37,-28,-22,-20,-21,-26,-34,-44,-54,-63,-63,-57,-47,-37,-28,-22,-20,-21,-26,-34,-44,-54,-63,-63,-57,-47,-37,-28,-22,-20,-21,-26,-34,-44,-54,-63,-63,-57,-47,-37,-28,-22,-20,-21,-26,-34,-41.5,-41.5];
      | D=[190,160,150,140,130,123,110,100,90,80,50,50,49,44,37,31,25,21,20,21,24,24,28,30,29,26,20,14,7,2,-2,-4,-3,1,1,4,6,6,2,-3,-9,-16,-22,-25,-27,-26,-22,-22,-19,-17,-18,-21,-26,-33,-39,-45,-49,-50,-70];
      | plot(C,D);
      | 
      | 
      | %load figure -120deg
      | c=1*exp(sqrt(-1)*(-60*pi/180));
      | l=A1+j*B1;
      | m=l*c;
      | E=real(m);F=imag(m);
      | E=E+34.4400;F=F-118.53;
      | plot(E,F);
      | 
      | %load figure +120deg
      | c=1*exp(sqrt(-1)*(60*pi/180));
      | l=A+j*B;
      | m=l*c;
      | G=real(m);
      | H=imag(m);
      | G=G-117.44;H=H-118.5300;
      | plot(G,H);
      | 
      | color('black');
      | port_label('LConn', 1, 'A')
      | port_label('LConn', 2, 'B')
      | port_label('LConn', 3, 'C')
  675 Yg Z : spsThreePhaseSeriesRLCLoadLib/Three-Phase Series RLC Load  LConnTagsString=A|B|C  Configuration=Y (grounded)  NominalVoltage=[ 1.021 1.042 1.0174]*2401.78  Vabc=[ 1.0 1.0 1.0]*2401.78  Vabcp=[1e3 1e3 1e3]  NominalFrequency=60  UnbalancedPower=on  ActivePower="[17 66  117]*1e3/2"  InductivePower="[10 38  68]*1e3/2"  CapacitivePower=100  Pabc=[0 0 0]  QLabc=[0 0 0]  QCabc=[200 200 200]*1e3*a  Pabcp=[10e3 9e3 11e3]  QLabcp=[100 90 110]  QCabcp=[100 90 110]  Measurements=None  LoadType=constant Z
  680 : Subsystem
  684 : Subsystem
  692 : spsThreePhaseVIMeasurementLib/Three-Phase V-I Measurement  VoltageMeasurement=phase-to-ground  SetLabelV=on  LabelV=V692  Vpu=off  VpuLL=off  CurrentMeasurement=no  SetLabelI=on  LabelI=I634  Ipu=off  Pbase=100e6  Vbase=24900  OutputType=Complex  PhasorSimulation=off  PSBequivalent=0
  692 D I : Subsystem  mask(Three Phase Delta ZIP Load (Phasor)){Vnom=4160, fnom=60, Pnom=[1e-6 1e-6 170 ]*1e3*a, Qnom=[0 0 151]*1e3*a, LoadType=Constant I, Vlim=0.7}
      mask prompts: Vnom "Nominal Ph-Ph Voltage (Vrms)"; fnom "Nominal Frequency fn (Hz)"; Pnom "Nominal Per Phase Active Power [Pab Pbc Pca] (W)"; Qnom "Nominal Per Phase Reactive Power [Qab Qbc Qca] (VAR)"; LoadType "Load Type"; Vlim "Minimum Voltage (pu)"
      mask help:
      | Notes:
      | Three Phase Delta Connected ZIP load model which gets converted to constant Z type if the voltage becomes lower than the "Minimum voltage".
      mask TypeOptions LoadType: Constant Z | Constant I | Constant P
      mask DialogControl ParameterTabVar0 Prompt: Parameters
      mask DialogControl ParameterTabVar01 Prompt: Type
      mask Display:
      | color('red');
      | %load figure 0deg
      | A=[-210,-180,-170,-160,-147,-140,-130,-120,-110,-80,-50,-49,-45,-39,-33,-26,-21,-18,-17,-19,-22,-22,-26,-27,-25,-22,-16,-9,-3,2,6,6,4,1,1,-3,-4,-2,2,7,14,20,26,29,30,28,24,24,21,20,21,25,31,37,44,49,50,50,80];
      | B=[-41.5,-41.5,-63,-20,-63,-20,-63,-20,-41.5,-41.5,-41.5,-34,-26,-21,-20,-22,-28,-37,-47,-57,-63,-63,-54,-44,-34,-26,-21,-20,-22,-28,-37,-47,-57,-63,-63,-54,-44,-34,-26,-21,-20,-22,-28,-37,-47,-57,-63,-63,-54,-44,-34,-26,-21,-20,-22,-28,-37,-41.50,-41.5];
      | plot(A,B);
      | 
      | %load figure 0deg inverted
      | A1=[-80,-50,-49,-45,-39,-33,-26,-21,-18,-17,-19,-22,-22,-26,-27,-25,-22,-16,-9,-3,2,6,6,4,1,1,-3,-4,-2,2,7,14,20,26,29,30,28,24,24,21,20,21,25,31,37,44,49,50,50,80,110,120,130,143,150,160,170,180,210];
      | B1=[-41.5,-41.5,-34,-26,-21,-20,-22,-28,-37,-47,-57,-63,-63,-54,-44,-34,-26,-21,-20,-22,-28,-37,-47,-57,-63,-63,-54,-44,-34,-26,-21,-20,-22,-28,-37,-47,-57,-63,-63,-54,-44,-34,-26,-21,-20,-22,-28,-37,-41.5,-41.5,-41.5,-63,-20,-63,-20,-63,-20,-41.5,-41.5];
      | 
      | 
      | %load figure -120deg
      | c=1*exp(sqrt(-1)*(-60*pi/180));
      | l=A1+j*B1;
      | m=l*c;
      | E=real(m);F=imag(m);
      | E=E+10.94;F=F+161.1;
      | plot(E,F);
      | 
      | %load figure +120deg
      | c=1*exp(sqrt(-1)*(60*pi/180));
      | l=A1+j*B1;
      | m=l*c;
      | G=real(m);
      | H=imag(m);
      | G=G-205.94;H=H+48.53;
      | plot(G,H);
      | 
      | color('black');
      | port_label('LConn', 1, 'A')
      | port_label('LConn', 2, 'B')
      | port_label('LConn', 3, 'C')
  692-675 606 : spsThreePhasePISectionLineLib/Three-Phase PI Section Line  LConnTagsString=a|b|c  RConnTagsString=A|B|C  Length=500*ft2km  Frequency=60  Resistances=[R1_606 R0_606]  Inductances=[L1_606 L0_606]  Capacitances=[C1_606 C0_606]
  BUS 684 a : spsVoltageMeasurementLib/Voltage Measurement  PhasorSimulation=off  OutputType=Complex  PSBequivalent=0
  BUS 684 b : spsVoltageMeasurementLib/Voltage Measurement  PhasorSimulation=off  OutputType=Complex  PSBequivalent=0
  Breaker{,1..4} (5 alike) : spsBreakerLib/Breaker  InitialState=0  SwitchingTimes="[1/60  5/60]"  External=on  BreakerResistance=0.01  SnubberResistance=1e6  SnubberCapacitance=inf  Measurements=None  MoreParameters=on  NoBreakLoop=off
  Bus 611 : spsVoltageMeasurementLib/Voltage Measurement  PhasorSimulation=off  OutputType=Complex  PSBequivalent=0
  Bus {632..634,650,671,675,680,692} (8 alike) : spsThreePhaseVIMeasurementLib/Three-Phase V-I Measurement  VoltageMeasurement=phase-to-ground  SetLabelV=off  LabelV=Vabc  Vpu=off  VpuLL=off  CurrentMeasurement=yes  SetLabelI=off  LabelI=Iabc  Ipu=off  Pbase=100e6  Vbase=500e3  OutputType=Complex  PhasorSimulation=off  PSBequivalent=0
  Bus 645 : Mux  Inputs=2
  Bus 645 b : spsVoltageMeasurementLib/Voltage Measurement  PhasorSimulation=off  OutputType=Complex  PSBequivalent=0
  Bus 645 c : spsVoltageMeasurementLib/Voltage Measurement  PhasorSimulation=off  OutputType=Complex  PSBequivalent=0
  Bus 646 : Mux  Inputs=2
  Bus 646 b : spsVoltageMeasurementLib/Voltage Measurement  PhasorSimulation=off  OutputType=Complex  PSBequivalent=0
  Bus 646 c : spsVoltageMeasurementLib/Voltage Measurement  PhasorSimulation=off  OutputType=Complex  PSBequivalent=0
  Bus 652 : spsVoltageMeasurementLib/Voltage Measurement  PhasorSimulation=off  OutputType=Complex  PSBequivalent=0
  Bus 684 : Mux  Inputs=2
  Current Measurement{,1..7} (8 alike) : spsCurrentMeasurementLib/Current Measurement  PhasorSimulation=off  OutputType=Complex  PSBequivalent=0
  Display : Display
  Ground{,1..10,12} (12 alike) : spsGroundLib/Ground  LConnTagsString=a
  Mux : Mux  Inputs=12
  Node Voltages : Subsystem
  PV_POWER : Sum  Inputs=|+++
  Power (3ph, Phasor){,1..7} (8 alike) : spsPower3phPhasorLib/Power (3ph, Phasor)
      settings: LibrarySourceBlock=|
      | sps_lib/Sensors and Measurements/Power
      | (3ph, Phasor)
  Product{,1..7} (8 alike) : Product
  RG60in : spsThreePhaseVIMeasurementLib/Three-Phase V-I Measurement  VoltageMeasurement=phase-to-ground  SetLabelV=on  LabelV=RG60in  Vpu=off  VpuLL=off  CurrentMeasurement=yes  SetLabelI=on  LabelI=IRG60in  Ipu=off  Pbase=100e6  Vbase=24900  OutputType=Complex  PhasorSimulation=off  PSBequivalent=0
  RG60out : spsThreePhaseVIMeasurementLib/Three-Phase V-I Measurement  VoltageMeasurement=phase-to-ground  SetLabelV=on  LabelV=RG60out  Vpu=off  VpuLL=off  CurrentMeasurement=yes  SetLabelI=on  LabelI=IRG60out  Ipu=off  Pbase=100e6  Vbase=24900  OutputType=Complex  PhasorSimulation=off  PSBequivalent=0
  Regulator 1 : Subsystem
  "Regulator Taps " : Subsystem
  Scope{,1..11,611} (13 alike) : Scope
      Scope settings: ActiveDisplayYMinimum=-4245.7873  ActiveDisplayYMaximum=4245.7873
      Scope1 settings: ActiveDisplayYMinimum=-9561.1332  ActiveDisplayYMaximum=8552.7863  DataLoggingVariableName=ScopeData3
      Scope10 settings: ActiveDisplayYMinimum=-9472.9882  ActiveDisplayYMaximum=8516.5104  DataLoggingVariableName=ScopeData13
      Scope11 settings: ActiveDisplayYMinimum=-9640.0894  ActiveDisplayYMaximum=8730.2364  DataLoggingVariableName=ScopeData14
      Scope2 settings: ActiveDisplayYMinimum=-9345.5123  ActiveDisplayYMaximum=9079.6398  DataLoggingVariableName=ScopeData4
      Scope3 settings: ActiveDisplayYMinimum=-1302.0011  ActiveDisplayYMaximum=1984.2082  DataLoggingVariableName=ScopeData5
      Scope4 settings: ActiveDisplayYMinimum=-8125.797  ActiveDisplayYMaximum=7480.0067  DataLoggingVariableName=ScopeData6
      Scope5 settings: ActiveDisplayYMinimum=-8090.3636  ActiveDisplayYMaximum=7502.4289  DataLoggingVariableName=ScopeData7
      Scope6 settings: ActiveDisplayYMinimum=-8090.3735  ActiveDisplayYMaximum=7502.45  DataLoggingVariableName=ScopeData8
      Scope611 settings: ActiveDisplayYMinimum=-7167.4602  ActiveDisplayYMaximum=6529.3364  DataLoggingVariableName=ScopeData11
      Scope7 settings: ActiveDisplayYMinimum=-8399.7354  ActiveDisplayYMaximum=8269.5642  DataLoggingVariableName=ScopeData9
      Scope8 settings: ActiveDisplayYMinimum=-7900.2078  ActiveDisplayYMaximum=8327.1331  DataLoggingVariableName=ScopeData10
      Scope9 settings: Title=Bus 684  ActiveDisplayYMinimum=-9863.3724  ActiveDisplayYMaximum=23209.2775  DataLoggingVariableName=ScopeData12
  Substation Power : Subsystem
  Subsystem : Subsystem
  Subsystem611 : Subsystem
  Subsystem634 : Subsystem
  Subsystem645 : Subsystem
  Subsystem646 : Subsystem
  Subsystem652 : Subsystem
  Subsystem671 : Subsystem
  Subsystem675 : Subsystem
  Subsystem692 : Subsystem
  Sum : Sum  Inputs=|++++++++
  Sum1 : Sum  Inputs=|++
  Sum2 : Sum  Inputs=|++
  Sum3 : Sum  Inputs=|++
  Three-Phase Transformer (Two Windings) : spsThreePhaseTransformerTwoWindingsLib/Three-Phase Transformer (Two Windings)  Winding1Connection=Yg  Winding2Connection=Yg  CoreType=Three single-phase transformers  SetSaturation=off  Hysteresis=off  DataFile='hysteresis'  SetInitialFlux=off  Measurements=None  UNITS=pu  NominalPower=[ 500e3 , 60 ]  Winding1=[4160 0.011 0.02]  Winding2=[480 0 0]  Rm=500  Lm=500  L0=0.5  Saturation=[ 0,0 ; 0.0024,1.2 ; 1.0,1.52 ]  InitialFluxes=[ 0.8 , -0.8 , 0.7 ]  BreakLoop=off  DiscreteSolver=Trapezoidal iterative  DataType=off  TransfoNumber=1
  Three-Phase Breaker : spsThreePhaseBreakerLib/Three-Phase Breaker  InitialState=closed  SwitchA=off  SwitchB=off  SwitchC=off  SwitchTimes=50  External=off  BreakerResistance=0.0001  SnubberResistance=inf  SnubberCapacitance=0  Measurements=None
  Three-Phase Breaker{1..5} (5 alike) : spsThreePhaseBreakerLib/Three-Phase Breaker  InitialState=open  SwitchA=on  SwitchB=on  SwitchC=on  SwitchTimes="[1/60  5/60]"  External=on  BreakerResistance=0.01  SnubberResistance=1e6  SnubberCapacitance=inf  Measurements=None
  Three-Phase Source : spsThreePhaseSourceLib/Three-Phase Source  InternalConnection=Yg  VoltagePhases=on  Voltage=25e3  PhaseAngle=0  Voltage_phases=[ 1.0 1.0 1.0]*2401.78  PhaseAngles_phases=[0 -120 120]  Frequency=60  NonIdealSource=off  SpecifyImpedance=off  Resistance=.001  Inductance=16.58e-6  ShortCircuitLevel=100e6  BaseVoltage=4160  XRratio=7  BusType=swing  Pref=10e3  Qref=0  Prefabc=[10e3, 10e3, 10e3]  Qrefabc=[0, 0, 0]  Qmin=-inf  Qmax=inf
  To Workspace : ToWorkspace  VariableName=Psource_GA  SampleTime=-1
  To Workspace1 : ToWorkspace  VariableName=P_bus  SampleTime=-1
  XFXFM1 : spsThreePhaseVIMeasurementLib/Three-Phase V-I Measurement  VoltageMeasurement=phase-to-ground  SetLabelV=on  LabelV=XFXFM1  Vpu=off  VpuLL=off  CurrentMeasurement=no  SetLabelI=on  LabelI=I634  Ipu=off  Pbase=100e6  Vbase=24900  OutputType=Complex  PhasorSimulation=off  PSBequivalent=0
  powergui : spspowerguiLib/powergui  Priority=1  SimulationMode=Discrete  SampleTime=Ts  frequency=60  Iterations=50  frequencyindice=0  Pbase=100e6  ErrMax=1e-4  UnitsV=kV  UnitsW=MW  buscounter=0  FunctionMessages=off  echomessages=on  EnableUseOfTLC=off  CurrentSourceSwitches=off  DisableSnubberDevices=off  DisableRonSwitches=off  DisableVfSwitches=off  DisplayEquations=off  AutomaticDiscreteSolvers=off  SolverType=Tustin  Interpol=off  ExternalGateDelay=off  methode=off  Ts=0  x0status=blocks  SPID=off  SwTol=0  HookPort=off  NonlinearTolerance=1e-4  nMaxIteration=100  ContinueOnMaxIteration=off  RestoreLinks=warning  ResistiveCurrentMeasurement=off  Frange=[0:2:500]  Ylog=off  Xlog=on  ShowGrid=off  save=off  variable=ZData  structure=0  ZoomFFT=off  StartTime=0.0  cycles=1  DisplayStyle=1  fundamental=60  FreqAxis=off  MaxFrequency=1000  frequencyindicesteady=1  RmsSteady=1  display=off
  tag scope: Rg1=global
  wires:
  Regulator 1/1(Tap) -> [Rg1]
  Bus 632/1 -> "Power (3ph, Phasor)5"/1, Scope1/1
  Bus 633/1 -> "Power (3ph, Phasor)6"/1, Scope2/1
  Bus 634/1 -> "Power (3ph, Phasor)4"/1, Scope3/1
  Bus 675/1 -> "Power (3ph, Phasor)3"/1, Scope4/1
  Bus 692/1 -> "Power (3ph, Phasor)1"/1, Scope5/1
  Bus 671/1 -> Scope6/1, "Power (3ph, Phasor)2"/1
  Bus 680/1 -> "Power (3ph, Phasor)7"/1, Scope7/1
  Bus 652/1 -> Product3/1, Scope8/1
  Bus 611/1 -> Product2/2, Scope611/1
  Bus 684/1 -> Scope9/1
  BUS 684 a/1 -> Product7/2, Bus 684/1
  BUS 684 b/1 -> Product6/1, Bus 684/2
  Bus 645 c/1 -> Product5/2, Bus 645/2
  Bus 645/1 -> Scope10/1
  Bus 645 b/1 -> Product4/1, Bus 645/1
  Bus 646 c/1 -> Product1/2, Bus 646/2
  Bus 646/1 -> Scope11/1
  Bus 646 b/1 -> Product/2, Bus 646/1
  Bus 650/1 -> "Power (3ph, Phasor)"/1, Scope/1
  Bus 650/2 -> "Power (3ph, Phasor)"/2
  "Power (3ph, Phasor)"/1 -> To Workspace/1
  Mux/1 -> To Workspace1/1
  Sum1/1 -> Sum/1, Mux/1
  Sum2/1 -> Sum/2, Mux/2
  Product2/1 -> Sum/3, Mux/3
  Product3/1 -> Mux/4, Sum/4
  "Power (3ph, Phasor)1"/1 -> Mux/5
  "Power (3ph, Phasor)4"/1 -> Sum/6, Mux/6
  "Power (3ph, Phasor)3"/1 -> Sum/7, Mux/7
  "Power (3ph, Phasor)2"/1 -> Sum/8, Mux/8
  Subsystem634/1(Power) -> PV_POWER/1
  Subsystem671/1(Power) -> PV_POWER/2
  Subsystem675/1(Power) -> PV_POWER/3
  Current Measurement1/1 -> Product/1
  Current Measurement/1 -> Product1/1
  Product/1 -> Sum1/1
  Product1/1 -> Sum1/2
  Current Measurement2/1 -> Product2/1
  Current Measurement3/1 -> Product3/2
  Current Measurement4/1 -> Product4/2
  Current Measurement5/1 -> Product5/1
  Product4/1 -> Sum2/1
  Product5/1 -> Sum2/2
  Bus 692/2 -> "Power (3ph, Phasor)1"/2
  Bus 671/2 -> "Power (3ph, Phasor)2"/2
  Bus 675/2 -> "Power (3ph, Phasor)3"/2
  Bus 634/2 -> "Power (3ph, Phasor)4"/2
  PV_POWER/1 -> Subsystem/1(PV_Power)
  Sum/1 -> Display/1
  Subsystem/1(671) -> Three-Phase Breaker4/1, Three-Phase Breaker5/1
  Subsystem/2(634) -> Three-Phase Breaker3/1
  Subsystem/3(675) -> Three-Phase Breaker2/1
  Subsystem/4(692) -> Three-Phase Breaker1/1
  Subsystem/5(646) -> Breaker3/1, Breaker4/1
  Subsystem/6(645) -> Breaker2/1
  Subsystem/7(611) -> Breaker/1
  Subsystem/8(652) -> Breaker1/1
  Current Measurement6/1 -> Product6/2
  Current Measurement7/1 -> Product7/1
  Product7/1 -> Sum3/1
  Product6/1 -> Sum3/2
  Sum3/1 -> Mux/9
  Bus 632/2 -> "Power (3ph, Phasor)5"/2
  "Power (3ph, Phasor)5"/1 -> Mux/10
  Bus 633/2 -> "Power (3ph, Phasor)6"/2
  "Power (3ph, Phasor)6"/1 -> Mux/11
  Bus 680/2 -> "Power (3ph, Phasor)7"/2
  "Power (3ph, Phasor)7"/1 -> Mux/12
  connections:
  601abc/LConn2 -- Three-Phase Breaker5/LConn2 -- 671/RConn2 -- Bus 671/LConn2 -- Three-Phase Breaker/LConn2
  Current Measurement2/LConn1 -- 611/LConn1
  632-633 602/LConn2 -- 632-645 603/LConn1 -- Bus 632/LConn2 -- 632/RConn2 -- 632 Yg PQ/LConn2 -- Subsystem671/RConn2 -- 632-671 601/LConn2
  Bus 675/LConn2 -- Three-Phase Breaker2/RConn2 -- 675 Y PQ/LConn2 -- 675 Yg Z/LConn2
  632-645 603/LConn2 -- Bus 632/LConn3 -- 632/RConn3 -- 632-633 602/LConn3 -- 632 Yg PQ/LConn3 -- 632-671 601/LConn3 -- Subsystem671/RConn3
  675 Yg Z/LConn3 -- Bus 675/LConn3 -- 675 Y PQ/LConn3 -- Three-Phase Breaker2/RConn3
  645/RConn1 -- Subsystem645/RConn1 -- 645Y PQ/LConn1 -- Breaker2/LConn1
  692 D I/LConn2 -- Three-Phase Breaker/RConn2 -- Three-Phase Breaker1/LConn2
  632-671 601/RConn3 -- 671/LConn3
  671/RConn1 -- Bus 671/LConn1 -- Three-Phase Breaker5/LConn1 -- 671-684 604/LConn1 -- 601abc/LConn1 -- Three-Phase Breaker/LConn1
  671/RConn3 -- Three-Phase Breaker5/LConn3 -- 671-684 604/LConn2 -- 601abc/LConn3 -- Three-Phase Breaker/LConn3 -- Bus 671/LConn3
  692/LConn3 -- Subsystem692/RConn3 -- Three-Phase Breaker1/RConn3
  692 D I/LConn1 -- Three-Phase Breaker1/LConn1 -- Three-Phase Breaker/RConn1
  632-633 602/LConn1 -- Subsystem671/RConn1 -- Bus 632/LConn1 -- 632/RConn1 -- 632-671 601/LConn1 -- 632 Yg PQ/LConn1
  Bus 675/LConn1 -- 675 Yg Z/LConn1 -- 675 Y PQ/LConn1 -- Three-Phase Breaker2/RConn1
  632-671 601/RConn2 -- 671/LConn2 -- Three-Phase Breaker4/LConn2
  671/LConn1 -- Three-Phase Breaker4/LConn1 -- Three-Phase Breaker4/LConn3 -- 632-671 601/RConn1
  692/RConn3 -- Bus 692/LConn3 -- 692-675 606/LConn3
  633/LConn2 -- 632-633 602/RConn2
  Bus 634/LConn3 -- Three-Phase Breaker3/LConn3 -- 634/RConn3
  645-646 603/RConn1 -- Subsystem646/RConn1 -- 646/RConn1
  XFXFM1/RConn2 -- Subsystem634/RConn2 -- 634/LConn2
  650/LConn1 -- Three-Phase Source/RConn1
  633/LConn1 -- 632-633 602/RConn1
  692/RConn2 -- 692-675 606/LConn2 -- Bus 692/LConn2
  680/RConn1 -- Bus 680/LConn1 -- 601abc/RConn1
  Regulator 1/LConn2 -- RG60in/RConn2
  692-675 606/RConn2 -- Subsystem675/RConn2 -- 675/LConn2
  645-646 603/RConn2 -- 646/RConn2 -- Subsystem646/RConn2
  633/RConn3 -- Bus 633/LConn3 -- Three-Phase Transformer (Two Windings)/LConn3
  Regulator 1/RConn3 -- RG60out/LConn3
  Regulator 1/RConn2 -- RG60out/LConn2
  XFXFM1/LConn2 -- Three-Phase Transformer (Two Windings)/RConn2
  632-645 603/RConn2 -- Subsystem645/RConn2 -- 645/RConn2
  684/LConn1 -- BUS 684 a/LConn1 -- 607a/LConn1
  650-632 601/RConn2 -- 632/LConn2
  650/LConn3 -- Three-Phase Source/RConn3
  Bus 634/LConn2 -- 634/RConn2 -- Three-Phase Breaker3/LConn2
  650-632 601/RConn3 -- 632/LConn3
  605c/LConn1 -- BUS 684 b/LConn1 -- 684/LConn2
  652Y Z/RConn1 -- Ground1/LConn1
  Bus 645 c/LConn1 -- 645-646 603/LConn2 -- Current Measurement5/RConn1
  Regulator 1/LConn3 -- RG60in/RConn3
  605c/RConn1 -- Subsystem611/RConn1 -- 611/RConn1
  650-632 601/RConn1 -- 632/LConn1
  680/RConn2 -- Bus 680/LConn2 -- 601abc/RConn2
  692/RConn1 -- Bus 692/LConn1 -- 692-675 606/LConn1
  XFXFM1/RConn3 -- Subsystem634/RConn3 -- 634/LConn3
  633/RConn1 -- Bus 633/LConn1 -- Three-Phase Transformer (Two Windings)/LConn1
  Regulator 1/RConn1 -- RG60out/LConn1
  675/LConn3 -- Subsystem675/RConn3 -- 692-675 606/RConn3
  Bus 634/LConn1 -- 634/RConn1 -- Three-Phase Breaker3/LConn1
  650-632 601/LConn3 -- RG60out/RConn3
  611Y I/RConn1 -- Ground3/LConn1
  Bus 652/LConn1 -- Current Measurement3/LConn1 -- 652/LConn1
  650/LConn2 -- Three-Phase Source/RConn2
  Bus 645 b/LConn1 -- 645-646 603/LConn1 -- Current Measurement4/RConn1
  652/RConn1 -- Subsystem652/RConn1 -- 607a/RConn1
  650-632 601/LConn1 -- RG60out/RConn1
  XFXFM1/LConn1 -- Three-Phase Transformer (Two Windings)/RConn1
  645Y PQ/RConn1 -- Ground/LConn1
  Bus 646 b/LConn1 -- Breaker3/LConn1 -- Current Measurement1/LConn1
  Regulator 1/LConn1 -- RG60in/RConn1
  680/RConn3 -- Bus 680/LConn3 -- 601abc/RConn3
  650-632 601/LConn2 -- RG60out/RConn2
  Ground2/LConn1 -- 611 Z/RConn1
  XFXFM1/LConn3 -- Three-Phase Transformer (Two Windings)/RConn3
  RG60in/LConn1 -- Bus 650/LConn1 -- 650/RConn1
  XFXFM1/RConn1 -- Subsystem634/RConn1 -- 634/LConn1
  633/RConn2 -- Bus 633/LConn2 -- Three-Phase Transformer (Two Windings)/LConn2
  650/RConn2 -- RG60in/LConn2 -- Bus 650/LConn2
  Bus 646 c/LConn1 -- Current Measurement/RConn1 -- 646 Z/RConn1
  633/LConn3 -- 632-633 602/RConn3
  692-675 606/RConn1 -- Subsystem675/RConn1 -- 675/LConn1
  RG60in/LConn3 -- Bus 650/LConn3 -- 650/RConn3
  Bus 652/LConn2 -- Ground12/LConn1
  Bus 611/LConn2 -- Ground4/LConn1
  BUS 684 a/LConn2 -- Ground5/LConn1
  BUS 684 b/LConn2 -- Ground6/LConn1
  Bus 645 b/LConn2 -- Ground7/LConn1
  Bus 646 b/LConn2 -- Ground8/LConn1
  Bus 645 c/LConn2 -- Ground9/LConn1
  Bus 646 c/LConn2 -- Ground10/LConn1
  Current Measurement/LConn1 -- Breaker4/LConn1
  646 Z/LConn1 -- Current Measurement1/RConn1
  Bus 611/LConn1 -- Current Measurement2/RConn1 -- Breaker/LConn1
  Breaker1/LConn1 -- Current Measurement3/RConn1
  645/LConn1 -- Current Measurement4/LConn1
  Current Measurement5/LConn1 -- 645/LConn2
  611Y I/LConn1 -- Breaker/RConn1 -- 611 Z/LConn1
  652Y Z/LConn1 -- Breaker1/RConn1
  632-645 603/RConn1 -- Breaker2/RConn1
  692/LConn1 -- Subsystem692/RConn1 -- Three-Phase Breaker1/RConn1
  692 D I/LConn3 -- Three-Phase Breaker1/LConn3 -- Three-Phase Breaker/RConn3
  692/LConn2 -- Subsystem692/RConn2 -- Three-Phase Breaker1/RConn2
  Breaker3/RConn1 -- 646/LConn1
  Breaker4/RConn1 -- 646/LConn2
  675/RConn3 -- Three-Phase Breaker2/LConn3
  675/RConn2 -- Three-Phase Breaker2/LConn2
  675/RConn1 -- Three-Phase Breaker2/LConn1
  634 Yg PQ/LConn3 -- Three-Phase Breaker3/RConn3
  Three-Phase Breaker3/RConn2 -- 634 Yg PQ/LConn2
  634 Yg PQ/LConn1 -- Three-Phase Breaker3/RConn1
  671 Yg PQ/LConn3 -- Three-Phase Breaker4/RConn3
  671 Yg PQ/LConn2 -- Three-Phase Breaker4/RConn2
  Three-Phase Breaker4/RConn1 -- 671 Yg PQ/LConn1
  671 D PQ/LConn1 -- Three-Phase Breaker5/RConn1
  Three-Phase Breaker5/RConn2 -- 671 D PQ/LConn2
  Three-Phase Breaker5/RConn3 -- 671 D PQ/LConn3
  671-684 604/RConn2 -- Current Measurement6/LConn1
  Current Measurement6/RConn1 -- 684/RConn2
  Current Measurement7/RConn1 -- 684/RConn1
  Current Measurement7/LConn1 -- 671-684 604/RConn1
